simulink model "pend_linear"  (R2025a)
settings: Solver=ode1  StartTime=0.0  StopTime=30  FixedStep=0.001  RelTol=1e-3
values from neighbouring files (symbols this model uses):
  g = 9.81    [lyapunov_analysis.m]
  l = 1.5    [lyapunov_analysis.m]
  m = 0.2    [lyapunov_analysis.m]
  M = 4    [lyapunov_analysis.m]
  s = size(K_lqr)    [lyapunov_analysis.m]
undefined symbols (not defined in the file or in its folder): X, Y, Z
libraries: sm_lib x8, nesl_utility x6
settings Model: Creator=musta  LastModifiedBy=musta
settings ExplorerConfigSet: InternalSimMechanicsExplorerSettings=|
  | <ExplorerConfiguration>
  | 
  |   <canonicalview>default</canonicalview>
  | 
  |   <TilePanel>
  |     <TileInfo>
  |       <Tiles Columns="1" Count="1" Height="658" Rows="1" Width="1082">
  |         <Row Weight="1"/>
  |         <Column Weight="1"/>
  |         <Tile Height="1" Width="1" X="0" Y="0"/>
  |       </Tiles>
  |     </TileInfo>
  |     <SceneInfo>
  |       <SceneViewer>
  |         <IsThisViewStd>
  |           <IsStandardView>off</IsStandardView>
  |           <StandardViewName>Front</StandardViewName>
  |         </IsThisViewStd>
  |         <BGColor>
  |           <R>1</R>
  |           <G>1</G>
  |           <B>1</B>
  |           <A>1</A>
  |         </BGColor>
  |         <Camera>
  |           <DoPerspective>off</DoPerspective>
  |           <Position>
  |             <X>-125.80838194993663</X>
  |             <Y>-31.389791847607604</Y>
  |             <Z>-18.856914019622597</Z>
  |           </Position>
  |           <Center>
  |             <X>1.9892680500633659</X>
  |             <Y>0.098128152392395585</Y>
  |             <Z>0.22245598037740155</Z>
  |           </Center>
  |           <Up>
  |             <X>0.10963862506818191</X>
  |             <Y>-0.80132524097865632</Y>
  |             <Z>0.58809627618584437</Z>
  |           </Up>
  |           <XLim>1.6712452292347915</XLim>
  |           <YLim>1.6712452292347915</YLim>
  |           <ViewLimDist>0.01</ViewLimDist>
  |         </Camera>
  |       </SceneViewer>
  |     </SceneInfo>
  |   </TilePanel>
  | 
  |   <MechEditorPanel>
  |     <GfxPanelCameraMap/>
  |     <Cameras/>
  |     <VideoCreator>
  |       <IncludeTiles>All</IncludeTiles>
  |       <IncludeTime>on</IncludeTime>
  |       <IncludeWorldFrame>off</IncludeWorldFrame>
  |       <PlaybackSpeedRatio>1</PlaybackSpeedRatio>
  |       <FrameRate>30</FrameRate>
  |       <FrameSize>auto</FrameSize>
  |       <VideoFormat>UncompressedAVI</VideoFormat>
  |     </VideoCreator>
  |   </MechEditorPanel>
  | 
  |   <PlaybackSettings>
  |     <PlaybackSpeedFactor>16</PlaybackSpeedFactor>
  |   </PlaybackSettings>
  | 
  | </ExplorerConfiguration>

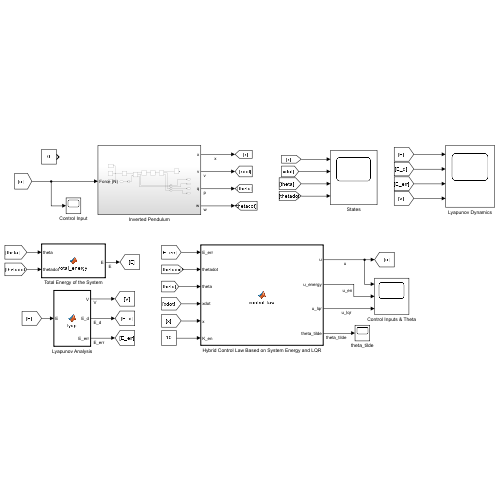
[thumbnail: Simulink's stored preview of the top-level diagram]
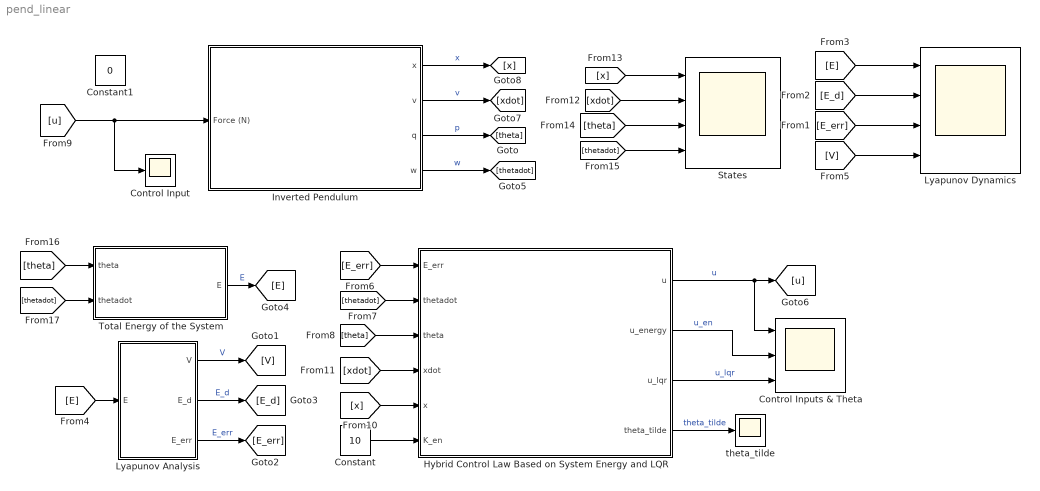
== system pend_linear ==
  Constant : Constant  Value=10
  Constant1 : Constant  Value=0
  Control Input : Scope
      settings: ActiveDisplayYMinimum=-19.200544394930702  ActiveDisplayYMaximum=9.6999990944749772
  Control Inputs & Theta : Scope  NumInputPorts=3
      settings: ActiveDisplayYMinimum=-1050.4109000019846  ActiveDisplayYMaximum=855.96481828984986  DataLoggingVariableName=ScopeData3
  Hybrid Control Law Based on System Energy and LQR : MATLAB Function  TreatAsAtomicUnit=on  SystemSampleTime=0.001
  Inverted Pendulum : Subsystem
  Lyapunov Analysis : MATLAB Function  TreatAsAtomicUnit=on
  Lyapunov Dynamics : Scope  NumInputPorts=4
      settings: ActiveDisplayYMinimum=-8.082141715030712  ActiveDisplayYMaximum=9.7503433268919757  DataLoggingVariableName=ScopeData2
  States : Scope  NumInputPorts=4
      settings: ActiveDisplayYMinimum=-62.753808076606532  ActiveDisplayYMaximum=75.993181608550685
  Total Energy of the System : MATLAB Function  TreatAsAtomicUnit=on
  theta_tilde : Scope
      settings: ActiveDisplayYMinimum=-4.1055457670697173  ActiveDisplayYMaximum=4.1399275305666361  DataLoggingVariableName=ScopeData4
  wires:
  Inverted Pendulum/1(x) -> [x]  "x"
  Inverted Pendulum/3(q) -> [theta]  "p"
  Inverted Pendulum/4(w) -> [thetadot]  "w"
  Total Energy of the System/1(E) -> [E]  "E"
  [E] -> Lyapunov Dynamics/1
  [E_d] -> Lyapunov Dynamics/2
  [E_err] -> Lyapunov Dynamics/3
  [V] -> Lyapunov Dynamics/4
  [E_err] -> Hybrid Control Law Based on System Energy and LQR/1(E_err)
  [thetadot] -> Hybrid Control Law Based on System Energy and LQR/2(thetadot)
  [theta] -> Hybrid Control Law Based on System Energy and LQR/3(theta)
  Hybrid Control Law Based on System Energy and LQR/1(u) -> Control Inputs & Theta/1, [u]  "u"
  [xdot] -> Hybrid Control Law Based on System Energy and LQR/4(xdot)
  [x] -> Hybrid Control Law Based on System Energy and LQR/5(x)
  Constant/1 -> Hybrid Control Law Based on System Energy and LQR/6(K_en)
  [u] -> Inverted Pendulum/1(Force (N)), Control Input/1
  Hybrid Control Law Based on System Energy and LQR/2(u_energy) -> Control Inputs & Theta/2  "u_en"
  Hybrid Control Law Based on System Energy and LQR/3(u_lqr) -> Control Inputs & Theta/3  "u_lqr"
  Inverted Pendulum/2(v) -> [xdot]  "v"
  [xdot] -> States/2
  [x] -> States/1
  [theta] -> States/3
  [thetadot] -> States/4
  [theta] -> Total Energy of the System/1(theta)
  [thetadot] -> Total Energy of the System/2(thetadot)
  Hybrid Control Law Based on System Energy and LQR/4(theta_tilde) -> theta_tilde/1  "theta_tilde"
  [E] -> Lyapunov Analysis/1(E)
  Lyapunov Analysis/2(E_d) -> [E_d]  "E_d"
  Lyapunov Analysis/1(V) -> [V]  "V"
  Lyapunov Analysis/3(E_err) -> [E_err]  "E_err"

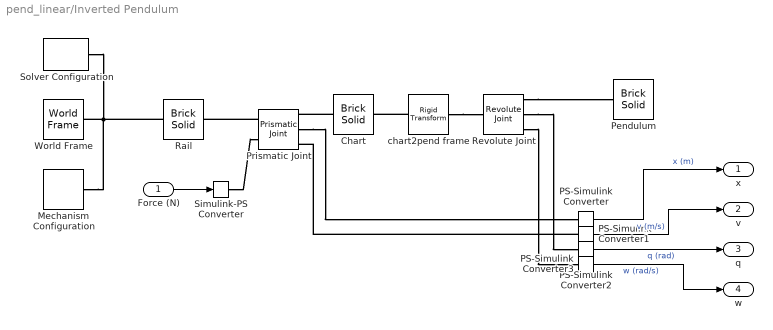
== system pend_linear/Inverted Pendulum ==
  Force (N) : Inport
  Chart : sm_lib/Body Elements/Brick Solid  BrickDimensions=[2 1 1]  BrickDimensionsUnits=m  ExportEntireGeometry=off  InertiaType=CalculateFromGeometry  BasedOnType=Mass  Density=1000  DensityUnits=kg/m^3  Mass=M  MassUnits=kg  CenterOfMass=[0 0 0]  CenterOfMassUnits=m  MomentsOfInertia=[8 2 3]  MomentsOfInertiaUnits=kg*m^2  ProductsOfInertia=[0 0 0]  ProductsOfInertiaUnits=kg*m^2  GraphicType=FromGeometry  MarkerShape=Sphere  MarkerSize=10  GraphicVisPropType=SimpleVisualProperties  GraphicDiffuseColor=[0.4 0.8 0.5]  GraphicOpacity=1  GraphicSpecularColor=[0.5 0.5 0.5 1.0]  GraphicAmbientColor=[0.15 0.15 0.15 1.0]  GraphicEmissiveColor=[0.0 0.0 0.0 1.0]  GraphicShininess=75  DoExposeReferenceFrame=on  SerializedFrames=|
      | <Frames>
      | 
      |   <Frame>
      |     <Id>Frame1</Id>
      |     <Value>
      |       <Name>rail</Name>
      |       <Origin>
      |         <Source>ReferenceFrame</Source>
      |         <FeatureName></FeatureName>
      |       </Origin>
      |       <PrimaryAxis>
      |         <DefinedDirection>+X</DefinedDirection>
      |         <Source>ReferenceFrame</Source>
      |         <SourceDirection>+Z</SourceDirection>
      |         <FeatureName></FeatureName>
      |       </PrimaryAxis>
      |       <SecondaryAxis>
      |         <DefinedDirection>+Z</DefinedDirection>
      |         <Source>ReferenceFrame</Source>
      |         <SourceDirection>+X</SourceDirection>
      |         <FeatureName></FeatureName>
      |       </SecondaryAxis>
      |     </Value>
      |   </Frame>
      | 
      | </Frames>
  Mechanism Configuration : sm_lib/Utilities/Mechanism Configuration  UniformGravity=Constant  GravityVector=[0 0 -9.80665]  GravityVectorUnits=m/s^2  LinearizationDelta=0.001  JointModeTransitionNonlinearIterations=2
  PS-Simulink Converter{,1..3} (4 alike) : nesl_utility/PS-Simulink Converter  PhysicalDomain=network_engine_domain  SubClassName=ps_output  LeftPortType=input  RightPortType=output  PseudoPeriodic=off  Frequencies=[]  VectorFormat=inherit  Unit=inherit  AffineConversion=off
  Pendulum : sm_lib/Body Elements/Brick Solid  BrickDimensions=[0.4 0.4 3]  BrickDimensionsUnits=m  ExportEntireGeometry=off  InertiaType=CalculateFromGeometry  BasedOnType=Mass  Density=1000  DensityUnits=kg/m^3  Mass=m  MassUnits=kg  CenterOfMass=[0 0 0]  CenterOfMassUnits=m  MomentsOfInertia=[0.3 0.6 0.45]  MomentsOfInertiaUnits=kg*m^2  ProductsOfInertia=[0 0 0]  ProductsOfInertiaUnits=kg*m^2  GraphicType=FromGeometry  MarkerShape=Sphere  MarkerSize=10  GraphicVisPropType=SimpleVisualProperties  GraphicDiffuseColor=[0 0.2 0.4]  GraphicOpacity=1  GraphicSpecularColor=[0.5 0.5 0.5 1.0]  GraphicAmbientColor=[0.15 0.15 0.15 1.0]  GraphicEmissiveColor=[0.0 0.0 0.0 1.0]  GraphicShininess=75  DoExposeReferenceFrame=on  SerializedFrames=|
      | <Frames>
      | 
      |   <Frame>
      |     <Id>Frame1</Id>
      |     <Value>
      |       <Name>chart</Name>
      |       <Origin>
      |         <Source>GeometricFeature</Source>
      |         <FeatureName>+y -z curve</FeatureName>
      |       </Origin>
      |       <PrimaryAxis>
      |         <DefinedDirection>+Z</DefinedDirection>
      |         <Source>ReferenceFrame</Source>
      |         <SourceDirection>+Y</SourceDirection>
      |         <FeatureName></FeatureName>
      |       </PrimaryAxis>
      |       <SecondaryAxis>
      |         <DefinedDirection>+X</DefinedDirection>
      |         <Source>ReferenceFrame</Source>
      |         <SourceDirection>+X</SourceDirection>
      |         <FeatureName></FeatureName>
      |       </SecondaryAxis>
      |     </Value>
      |   </Frame>
      | 
      | </Frames>
  Prismatic Joint : sm_lib/Joints/Prismatic Joint  JointMode=Normal  CompositeWrenchDir=FollowerOnBase  CompositeWrenchFrame=BaseFrame  SenseConstraintForce=off  SenseConstraintTorque=off  SenseTotalForce=off  SenseTotalTorque=off  PositionTargetSpecify=off  PositionTargetPriority=High  PositionTargetValue=0  PositionTargetValueUnits=m  VelocityTargetSpecify=off  VelocityTargetPriority=High  VelocityTargetValue=0  VelocityTargetValueUnits=m/s  EquilibriumPosition=0  EquilibriumPositionUnits=m  SpringStiffness=0  SpringStiffnessUnits=N/m  DampingCoefficient=c  DampingCoefficientUnits=N/(m/s)  LowerLimitSpecify=off  LowerLimitBound=-1  LowerLimitBoundUnits=m  LowerLimitStiffness=1e6  LowerLimitStiffnessUnits=N/m  LowerLimitDamping=1e3  LowerLimitDampingUnits=N/(m/s)  LowerLimitTransitionRegionWidth=1e-4  LowerLimitTransitionRegionWidthUnits=m  UpperLimitSpecify=off  UpperLimitBound=1  UpperLimitBoundUnits=m  UpperLimitStiffness=1e6  UpperLimitStiffnessUnits=N/m  UpperLimitDamping=1e3  UpperLimitDampingUnits=N/(m/s)  UpperLimitTransitionRegionWidth=1e-4  UpperLimitTransitionRegionWidthUnits=m  TorqueActuationMode=InputTorque  MotionActuationMode=ComputedMotion  SensePosition=on  SenseVelocity=on  SenseAcceleration=off  SenseTorqueForce=off  SenseLowerLimitTorqueForce=off  SenseUpperLimitTorqueForce=off
  Rail : sm_lib/Body Elements/Brick Solid  BrickDimensions=[40 0.1 0.1]  BrickDimensionsUnits=m  ExportEntireGeometry=off  InertiaType=CalculateFromGeometry  BasedOnType=Density  Density=1000  DensityUnits=kg/m^3  Mass=1  MassUnits=kg  CenterOfMass=[0 0 0]  CenterOfMassUnits=m  MomentsOfInertia=[1 1 1]  MomentsOfInertiaUnits=kg*m^2  ProductsOfInertia=[0 0 0]  ProductsOfInertiaUnits=kg*m^2  GraphicType=FromGeometry  MarkerShape=Sphere  MarkerSize=10  GraphicVisPropType=SimpleVisualProperties  GraphicDiffuseColor=[0 0 0]  GraphicOpacity=1  GraphicSpecularColor=[0.5 0.5 0.5 1.0]  GraphicAmbientColor=[0.15 0.15 0.15 1.0]  GraphicEmissiveColor=[0.0 0.0 0.0 1.0]  GraphicShininess=75  DoExposeReferenceFrame=on  SerializedFrames=|
      | <Frames>
      | 
      |   <Frame>
      |     <Id>Frame1</Id>
      |     <Value>
      |       <Name>chart</Name>
      |       <Origin>
      |         <Source>ReferenceFrame</Source>
      |         <FeatureName></FeatureName>
      |       </Origin>
      |       <PrimaryAxis>
      |         <DefinedDirection>+X</DefinedDirection>
      |         <Source>ReferenceFrame</Source>
      |         <SourceDirection>+Z</SourceDirection>
      |         <FeatureName></FeatureName>
      |       </PrimaryAxis>
      |       <SecondaryAxis>
      |         <DefinedDirection>+Z</DefinedDirection>
      |         <Source>ReferenceFrame</Source>
      |         <SourceDirection>+X</SourceDirection>
      |         <FeatureName></FeatureName>
      |       </SecondaryAxis>
      |     </Value>
      |   </Frame>
      | 
      | </Frames>
  Revolute Joint : sm_lib/Joints/Revolute Joint  JointMode=Normal  CompositeWrenchDir=FollowerOnBase  CompositeWrenchFrame=BaseFrame  SenseConstraintForce=off  SenseConstraintTorque=off  SenseTotalForce=off  SenseTotalTorque=off  PositionTargetSpecify=on  PositionTargetPriority=High  PositionTargetValue=5  PositionTargetValueUnits=deg  VelocityTargetSpecify=on  VelocityTargetPriority=High  VelocityTargetValue=0  VelocityTargetValueUnits=deg/s  EquilibriumPosition=0  EquilibriumPositionUnits=deg  SpringStiffness=0  SpringStiffnessUnits=N*m/deg  DampingCoefficient=b  DampingCoefficientUnits=N*m*s/rad  LowerLimitSpecify=off  LowerLimitBound=-90  LowerLimitBoundUnits=deg  LowerLimitStiffness=1e4  LowerLimitStiffnessUnits=N*m/deg  LowerLimitDamping=10  LowerLimitDampingUnits=N*m/(deg/s)  LowerLimitTransitionRegionWidth=0.1  LowerLimitTransitionRegionWidthUnits=deg  UpperLimitSpecify=off  UpperLimitBound=90  UpperLimitBoundUnits=deg  UpperLimitStiffness=1e4  UpperLimitStiffnessUnits=N*m/deg  UpperLimitDamping=10  UpperLimitDampingUnits=N*m/(deg/s)  UpperLimitTransitionRegionWidth=0.1  UpperLimitTransitionRegionWidthUnits=deg  TorqueActuationMode=NoTorque  MotionActuationMode=ComputedMotion  SensePosition=on  SenseVelocity=on  SenseAcceleration=off  SenseTorqueForce=off  SenseLowerLimitTorqueForce=off  SenseUpperLimitTorqueForce=off
  Simulink-PS Converter : nesl_utility/Simulink-PS Converter  PhysicalDomain=network_engine_domain  SubClassName=ps_input  LeftPortType=input  RightPortType=output  PseudoPeriodic=off  Frequencies=[]  NoiseDistribution=none  NoiseParameters=[]  Unit=1  AffineConversion=off  FilteringAndDerivatives=provide  SimscapeFilterOrder=1  InputFilterTimeConstant=0.001  UdotUserProvided=0
  Solver Configuration : nesl_utility/Solver Configuration  PhysicalDomain=network_engine_domain  SubClassName=solver  LeftPortType=input  RightPortType=generic  Tones=[]  Harmonics=[]  SimulateNoise=off  Profile=off  UseLocalSampling=off  EnableSwitchedLinearOptims=on  FrequencyDomain=off  UseCCode=off  RelTol=0.001  AbsTol=0.001  MinStep=1e-09  ToWorkspace=off  RevertToSquareIcSolve=off  NumHomotopyIterations=100  PhasorMode=off  PhasorModeNumHarmonics=1  ConsistencySolver=NEWTON_XTOL_AFTER_FTOL  IndexReductionMethod=DerivativeReplacement  DoDC=off  ResidualTolerance=1e-09  ConsistencyTolSource=GLOBAL  ConsistencyAbsTol=0.001  ConsistencyRelTol=0.001  ConsistencyTolFactor=0.001  UseLocalSolver=off  LocalSolverChoice=NE_BACKWARD_EULER_ADVANCER  ResolveIndetEquations=on  FunctionEvalNumThread=1  LocalSolverSampleTime=0.001  DoFixedCost=off  MaxNonlinIter=3  MaxModeIter=2  ComputeImpulses=off  ImpulseIterations=2  LinearAlgebra=auto  LinearAlgebraNumThread=0  EquationFormulation=NE_TIME_EF  DelaysMemoryBudget=1024  AutomaticFiltering=on  FilteringTimeConstant=0.001  PartitionStorageMethod=AS_NEEDED  PartitionMemoryBudget=1024  PartitionMethod=ROBUST  MultibodyUseLocalSolver=off  MultibodyLocalSolverChoice=ODE1  MultibodyLocalSolverSampleTime=0.001
  World Frame : sm_lib/Frames and Transforms/World Frame
  chart2pend frame : sm_lib/Frames and Transforms/Rigid Transform  RotationMethod=StandardAxis  FollAlignAxisA=+X  BaseAlignAxisA=+Y  FollAlignAxisB=+Y  BaseAlignAxisB=+Z  RotationStandardAxis=+X  RotationAngle=90  RotationAngleUnits=deg  RotationArbitraryAxis=[0 0 1]  RotationSequenceAxes=FollowerAxes  RotationSequence=XYX  RotationSequenceAngles=[0 0 0]  RotationSequenceAnglesUnits=deg  RotationMatrix=[1 0 0;0 1 0;0 0 1]  Quaternion=[1 0 0 0]  TranslationMethod=Cartesian  TranslationCartesianOffset=[0 -0.9 0.5]  TranslationCartesianOffsetUnits=m  TranslationStandardAxis=+Y  TranslationStandardOffset=0.2  TranslationStandardOffsetUnits=m  TranslationROffset=0  TranslationROffsetUnits=m  TranslationThetaOffset=0  TranslationThetaOffsetUnits=deg  TranslationZOffset=0  TranslationZOffsetUnits=m
  x : Outport  VectorParamsAs1DForOutWhenUnconnected=off
  v : Outport  Port=2  VectorParamsAs1DForOutWhenUnconnected=off
  q : Outport  Port=3  VectorParamsAs1DForOutWhenUnconnected=off
  w : Outport  Port=4  VectorParamsAs1DForOutWhenUnconnected=off
  wires:
  PS-Simulink Converter1/1 -> v/1  "v (m/s)"
  PS-Simulink Converter/1 -> x/1  "x (m)"
  PS-Simulink Converter2/1 -> q/1  "q (rad)"
  PS-Simulink Converter3/1 -> w/1  "w (rad/s)"
  Force (N)/1 -> Simulink-PS Converter/1
  connections:
  Solver Configuration/RConn1 -- Mechanism Configuration/RConn1 -- Rail/RConn1 -- World Frame/RConn1
  chart2pend frame/RConn1 -- Revolute Joint/LConn1
  Chart/LConn1 -- Prismatic Joint/RConn1
  Revolute Joint/RConn1 -- Pendulum/LConn1
  chart2pend frame/LConn1 -- Chart/RConn1
  Prismatic Joint/LConn1 -- Rail/LConn1
  Prismatic Joint/RConn2 -- PS-Simulink Converter/LConn1
  Revolute Joint/RConn3 -- PS-Simulink Converter3/LConn1
  Simulink-PS Converter/RConn1 -- Prismatic Joint/LConn2
  Revolute Joint/RConn2 -- PS-Simulink Converter2/LConn1
  PS-Simulink Converter1/LConn1 -- Prismatic Joint/RConn3

== matlab function pend_linear/Lyapunov Analysis ==
  data: E input; V output; E_d output; m parameter; g parameter; l parameter; E_err output
function [V, E_d, E_err] = lyap(E, m, g, l)

E_d = 2*m*g*l;

V = 0.5*(E-E_d)^2;

E_err = E-E_d;

== matlab function pend_linear/Total Energy of the System ==
  data: theta input; E output; thetadot input; m parameter; g parameter; l parameter
function E = total_energy(theta, thetadot, m, g, l)

E = 0.5*m*l^2*thetadot^2 + m*g*l*(1-cos(theta));

== matlab function pend_linear/Hybrid Control Law Based on System Energy and LQR ==
  data: E_err input; u output; thetadot input; theta input; xdot input; x input; K_en input; u_energy output; u_lqr output; theta_tilde output; K_lqr parameter
function [u, u_energy, u_lqr, theta_tilde] = control_law(E_err, thetadot, theta, xdot, x, K_en, K_lqr)

% ---------- control law based on the energy ----------

u_energy = K_en*E_err*thetadot*cos(theta);

% ---------- control law based on LQR ----------

theta_tilde = theta-pi; % reference state


theta_tilde = atan2(sin(theta_tilde), cos(theta_tilde));
X = [x; xdot; theta_tilde; thetadot]; % state vector

u_lqr = -K_lqr*X; % LQR control law


% u_energy = max(min(u_energy,100), -100);
% u_lqr = max(min(u_lqr,20), -20);

% --------------------- combined control law ------------------------

persistent mode 

if isempty(mode)
    mode = 0; % mode 0 -> energy, mode 1-> LQR
end

theta_in = pi/12; % Enter LQR mode in ~20 degrees
theta_out = pi/9; % Keep LQR mode until ~30 degrees

beta = -20;
alpha = 1/(1+exp(-beta*(abs(theta_tilde)-theta_in)));


if mode == 0
    if abs(theta_tilde) <= theta_in 
        mode = 1;
    end
end

if mode == 1
    if abs(theta_tilde) >= theta_out
        mode = 0;
    end
end

if mode == 0
    u = u_energy;
else
    u = alpha*u_lqr + (1-alpha)*u_energy;
end
